simulink model "Team2_Final"  (R2023b)
settings: Solver=VariableStepAuto  StartTime=0.0  StopTime=30  RelTol=1e-3
libraries: commutil2 x3, commchan3 x2, simulink x2, commcnvcod2 x2, dspvision x2, commdigbbndpm3 x2, commfilt2 x2, dspquant2 x2, dspsnks4 x1, commsink2 x1, commrandsrc3 x1
settings Model: LastModifiedBy=bryan
settings OptimizationCC: BlockReduction=off  ConditionallyExecuteInputs=off
settings RTWCC: GPUComputeCapability=5.0

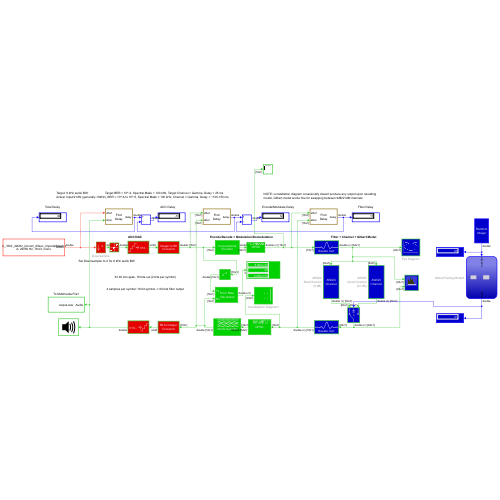
[thumbnail: Simulink's stored preview of the top-level diagram]
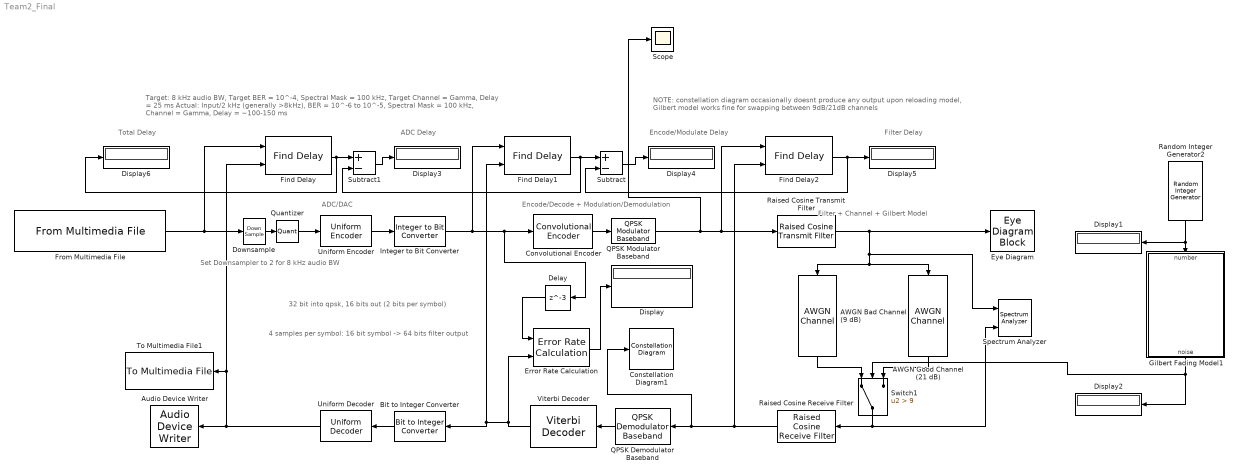
== system Team2_Final ==
  note: 4 samples per symbol: 16 bit symbol -> 64 bits filter output
  note: 32 bit into qpsk, 16 bits out (2 bits per symbol)
  note: Target: 8 kHz audio BW,                    Target BER = 10^-4, Spectral Mask = 100 kHz, Target Channel = Gamma, Delay = 25 ms
      | Actual: Input/2 kHz (generally >8kHz), BER = 10^-6 to 10^-5, Spectral Mask = 100 kHz, Channel = Gamma, Delay = ~100-150 ms
  note: NOTE: constellation diagram occasionally doesnt produce any output upon reloading model, Gilbert model works fine for swapping between 9dB/21dB channels
  note: Set Downsampler to 2 for 8 kHz audio BW
  note: Filter + Channel + Gilbert Model
  note: ADC/DAC
  note: Total Delay
  note: ADC Delay
  note: Encode/Modulate Delay
  note: Filter Delay
  note: Encode/Decode + Modulation/Demodulation
  AWGN Bad Channel (9 dB) : commchan3/AWGN Channel  LegacyMode=off  NoiseMethod="Signal to noise ratio  (SNR)"  noiseMode="Signal to noise ratio  (SNR)"  EbNo=9  EsNo=10  SNR=9  BitsPerSymbol=1  SignalPower=1  SamplesPerSymbol=1  SymbolPeriod=1  VarianceSource=Parameter  Variance=1  RandomStream=Global stream  Seed=67  SimulateUsing=Code generation
  AWGN Good Channel (21 dB) : commchan3/AWGN Channel  LegacyMode=off  NoiseMethod="Signal to noise ratio  (SNR)"  noiseMode="Signal to noise ratio  (SNR)"  EbNo=10  EsNo=10  SNR=21  BitsPerSymbol=1  SignalPower=1  SamplesPerSymbol=1  SymbolPeriod=1  VarianceSource=Parameter  Variance=1  RandomStream=Global stream  Seed=67  SimulateUsing=Code generation
  Audio Device Writer : dspsnks4/Audio Device Writer  Driver=DirectSound  Device=Default  InheritSampleRate=on  SampleRate=44100  BitDepth=16-bit integer  BufferSize=4096  NumBuffers=10  DefaultOutputChannelMapping=on  OutputChannelMapping=1:2  OutputNumUnderrunSamples=off  DriverIdx=1  DeviceWarnFlag=''
  Bit to Integer Converter : simulink/Logic and Bit Operations/Bit to Integer Converter  nbits=16  bitOrder=MSB first  signedOutputValues=Unsigned  outDtype=uint8  outDtypeSigned=Inherit via internal rule
  Constellation Diagram1 : ConstellationDiagram  WindowPosition=[931.000000,31.000000,600.000000,600.000000,]  Visible=on  ScopeFrameLocation=window
  Convolutional Encoder : commcnvcod2/Convolutional Encoder  trellis=poly2trellis(3,[6 7])  opMode=Continuous  DelayedResetAction=on  hasIniStPort=off  hasFinStPort=off  usePuncVector=off  punctureVector=[1; 1; 0; 1; 0; 1]  reset=Unused parameter value
      settings: LibrarySourceBlock=|
      | commhdlcnvcod/Convolutional
      | Encoder
  Delay : Delay  DelayLength=3  InitialCondition=0
  Display{,1..6} (7 alike) : Display
  Downsample : DownSample  RateOptions=Allow multirate processing
  Error Rate Calculation : commsink2/Error Rate Calculation  N=0  st_delay=48  cp_mode=Entire frame  subframe=[]  PMode=Port  WsName=ErrorVec  RsMode2=off  stop=off  numErr=100  maxBits=1e6
  Eye Diagram : EyeDiagramBlock  WindowPosition=[563.000000,200.000000,800.000000,500.000000,]  Visible=on  ScopeFrameLocation=window
  Find Delay : commutil2/Find Delay  corrLength=200  chgSigOP=off  stopUpdate=off  numConstDelay=3
  Find Delay1 : commutil2/Find Delay  corrLength=200  chgSigOP=off  stopUpdate=off  numConstDelay=3
  Find Delay2 : commutil2/Find Delay  corrLength=200  chgSigOP=off  stopUpdate=off  numConstDelay=3
  From Multimedia File : dspvision/From Multimedia File  inputFilename=C:\Users\bryan\Downloads\ELEC 391\Assignments\ELEC391_Sound_Files\Mono_16bit_22kHz_Uncom_60sec_ImperialMarch.wav  readRange=[1 Inf]  loop=on  numPlays=inf  outputStreams=Audio only  videoDataType=single  audioDataType=double  inheritSampleTime=on  userDefinedSampleTime=1/30  noAudioOutput=off  isIntensityVideo=off  fourcc=RGB  colorVideoFormat=Separate color signals  outputEOF=off  dataOrg=Column-major  audioFrameSize=1  computeAudioFrameSize=off  outSamplingMode=Sample based
      settings: LibrarySourceBlock=audiosources/From Multimedia File
  Gilbert Fading Model1 : Stateflow chart  TreatAsAtomicUnit=on
  Integer to Bit Converter : simulink/Logic and Bit Operations/Integer to Bit Converter  nbits=16  signedInputValues=Unsigned  bitOrder=MSB first  outDtype=double
  QPSK Demodulator Baseband : commdigbbndpm3/QPSK Demodulator Baseband  OutType=Bit  DecType=Hard decision  VarSource=Dialog  Variance=1  Dec=Gray  Ph=pi/4  outDtype1=Inherit via internal rule  outDtype2=Inherit via internal rule  derotateFactorWordLen=16  derotateFactorDataTypeStr=Inherit: Same word length as input  derotateFactorLastDataTypeStr=Inherit: Same word length as input
      settings: LibrarySourceBlock=|
      | commhdldigbbndpm/QPSK
      | Demodulator
      | Baseband
  QPSK Modulator Baseband : commdigbbndpm3/QPSK Modulator Baseband  InType=Bit  Enc=Gray  Ph=pi/4  outDtype=double  outWordLen=16  outUDDataType=sfix(16)  outFracLenMode=Best precision  outFracLen=15  outDataTypeStr=double  outLastDataTypeStr=double
      settings: LibrarySourceBlock=|
      | commhdldigbbndpm/QPSK
      | Modulator
      | Baseband
  Quantizer : Quantizer  QuantizationInterval=0.0625
  Raised Cosine Receive Filter : commfilt2/Raised Cosine Receive Filter  filtType=Square root  R=0.2  filtSpan=16  N=4  downFactor=4  downOffset=0  filterGain=1  InputProcessing=Columns as channels (frame based)  RateOptions=Enforce single-rate processing  framing=Mute  checkCoeff=off  variableName=rcRxFilt  currentFiltSpan=10  D=5  inputOffset=0  sampMode=Mute  saveAsFlag=0  rateMode=Downsampling  checkGain=Normalized  launchFVT=on  roundingMode=Floor  overflowMode=off  coeffDataTypeStr=Inherit: Same word length as input  coeffMin=[]  coeffMax=[]  coeffLastDataTypeStr=Inherit: Same word length as input  accumDataTypeStr=Inherit: Same as product output  accumLastDataTypeStr=Inherit: Same as product output  outputDataTypeStr=Inherit: Same as accumulator  outputMin=[]  outputMax=[]  outputLastDataTypeStr=Inherit: Same as accumulator
      settings: LibrarySourceBlock=|
      | commhdlfilt/Raised Cosine
      | Receive Filter
  Raised Cosine Transmit Filter : commfilt2/Raised Cosine Transmit Filter  filtType=Square root  R=0.2  filtSpan=16  N=4  filterGain=1  InputProcessing=Columns as channels (frame based)  RateOptions=Enforce single-rate processing  framing=Mute  checkCoeff=off  variableName=rcTxFilt  checkGain=Normalized  sampMode=Mute  saveAsFlag=0  currentFiltSpan=10  D=5  launchFVT=on  roundingMode=Floor  overflowMode=off  coeffDataTypeStr=Inherit: Same word length as input  coeffMin=[]  coeffMax=[]  coeffLastDataTypeStr=Inherit: Same word length as input  outputDataTypeStr=Inherit: Same as accumulator  outputMin=[]  outputMax=[]  outputLastDataTypeStr=Inherit: Same as accumulator
      settings: LibrarySourceBlock=|
      | commhdlfilt/Raised Cosine
      | Transmit Filter
  Random Integer Generator2 : commrandsrc3/Random Integer Generator  SetSize=101  SeedSource=Auto  Seed=0  SampleTime=1  SamplesPerFrame=1  OutputDataType=double  SimulateUsing=Interpreted execution
  Scope : Scope
  Spectrum Analyzer : SpectrumAnalyzer  NumInputPorts=2  WindowPosition=[622.000000,147.000000,960.000000,623.000000,]  Visible=on  ScopeFrameLocation=window  Span=128000  StartFrequency=-64000  StopFrequency=64000  YLimits=[-111.32557264,33.81595837]  ShowLegend=on  ExpandToolstrip=on
  Subtract : Sum  Inputs=+-
  Subtract1 : Sum  Inputs=+-
  Switch1 : Switch  Criteria=u2 > Threshold  Threshold=9  SaturateOnIntegerOverflow=off  InputSameDT=off
  To Multimedia File1 : dspvision/To Multimedia File  outputFilename=C:\Users\bryan\Downloads\ELEC 391\Assignments\output.wav  streamSelection=Audio only  videoCompressor=None (uncompressed)  audioCompressor=None (uncompressed)  imagePorts=One multidimensional signal  fileType=WAV  audioDatatype=16-bit integer  fourcc=RGB  videoQuality=75  mj2000CompFactor=10
      settings: LibrarySourceBlock=dspsnks4/To Multimedia File
  Uniform Decoder : dspquant2/Uniform Decoder  peak=1  bits=8  overflowMode=Saturate  otype=Double
  Uniform Encoder : dspquant2/Uniform Encoder  peak=1  bits=8  otype=Unsigned integer
  Viterbi Decoder : commcnvcod2/Viterbi Decoder  trellis=poly2trellis(3,[6 7])  isPunctured=off  punctureVector=[1; 1; 0; 1; 0; 1]  erasures=off  dectype=Hard decision  nsdecb=4  runSigValErrCheck=off  tbdepth=32  opmode=Continuous  reset=off  delayedResetAction=on  smWordLength=16  outDataType=double
      settings: LibrarySourceBlock=commhdlcnvcod/Viterbi Decoder
  wires:
  Downsample/1 -> Quantizer/1
  Quantizer/1 -> Uniform Encoder/1
  Uniform Encoder/1 -> Integer to Bit Converter/1
  Convolutional Encoder/1 -> QPSK Modulator Baseband/1
  QPSK Demodulator Baseband/1 -> Viterbi Decoder/1
  QPSK Modulator Baseband/1 -> Scope/1, Find Delay2/1, Raised Cosine Transmit Filter/1
  Raised Cosine Receive Filter/1 -> Find Delay2/2, Constellation Diagram1/1, QPSK Demodulator Baseband/1
  Uniform Decoder/1 -> Find Delay/2, To Multimedia File1/1, Audio Device Writer/1
  From Multimedia File/1 -> Find Delay/1, Downsample/1
  Error Rate Calculation/1 -> Display/1
  Viterbi Decoder/1 -> Error Rate Calculation/2, Find Delay1/2, Bit to Integer Converter/1
  Switch1/1 -> Raised Cosine Receive Filter/1, Spectrum Analyzer/2
  Integer to Bit Converter/1 -> Find Delay1/1, Delay/1, Convolutional Encoder/1
  Bit to Integer Converter/1 -> Uniform Decoder/1
  Delay/1 -> Error Rate Calculation/1
  Raised Cosine Transmit Filter/1 -> Eye Diagram/1, Spectrum Analyzer/1, AWGN Bad Channel (9 dB)/1, AWGN Good Channel (21 dB)/1
  AWGN Good Channel (21 dB)/1 -> Switch1/3
  AWGN Bad Channel (9 dB)/1 -> Switch1/1
  Gilbert Fading Model1/1(noise) -> Switch1/2, Display2/1
  Random Integer Generator2/1 -> Display1/1, Gilbert Fading Model1/1(number)
  Find Delay2/1 -> Subtract/2, Display5/1
  Find Delay1/1 -> Subtract1/2, Subtract/1
  Subtract/1 -> Display4/1
  Subtract1/1 -> Display3/1
  Find Delay/1 -> Subtract1/1, Display6/1

== stateflow chart Team2_Final/Gilbert Fading Model1 ==
  state Noise_Variance_BAD
    noise = 9;
  state Nosie_Variance_Good
    noise = 21;
  (default) -> Nosie_Variance_Good
  Noise_Variance_BAD -> Noise_Variance_BAD [order 1] : [number<=80]
  Nosie_Variance_Good -> Noise_Variance_BAD [order 1] : [number <=5]
  Nosie_Variance_Good -> Nosie_Variance_Good [order 2] : [number<=95]
  Noise_Variance_BAD -> Nosie_Variance_Good [order 2] : [number<=20]
  data: number input; noise output
